simulink model "CSI_0313_4DC"  (R2018a)
settings: Solver=FixedStepDiscrete  StartTime=0.0  StopTime=Tstop  FixedStep=Tdelt  MaxStep=1e-4  RelTol=1e-3
values from neighbouring files (symbols this model uses):
  C = 12e-6    (= 1.2e-05)    [Inputparameter.m]
  Cdc = 4.76*10^-3    (= 0.00476)    [Inputparameter.m]
  Cemc = 1.5e-6    (= 1.5e-06)    [Inputparameter.m]
  fanalog = 7000    [Run.m]
  fKIUdc = 6    [Run.m]
  fKPUdc = 0.4    [Run.m]
  fTs = Update/18000    (= 0.000111111111111)    [Run.m]
  K120 = 0.0    (= 0)    [Run.m]
  K21 = 0.0    (= 0)    [Run.m]
  K5 = 0.0    (= 0)    [Run.m]
  K7 = 0.0    (= 0)    [Run.m]
  Kipll = 1.0    (= 1)    [Run.m]
  klmt = 0.3    [Run.m]
  Kpll = 20.0    (= 20)    [Run.m]
  Lgrid = 7.717e-4*10    (= 0.007717)    [Run.m]
  Lline = 60e-6    (= 6e-05)    [Inputparameter.m]
  Lpwm = 184.8e-6    (= 0.0001848)    [Inputparameter.m]
  mode = 1    [Run.m]
  Nsw = 18000/fbase    [Run.m]
  Qbpf = 1.0    (= 1)    [Run.m]
  Rc = 10e-3    (= 0.01)    [Inputparameter.m]
  Remc = 1e-3    (= 0.001)    [Inputparameter.m]
  Rgrid = 2*pi*fbase*Lgrid/XR    [Run.m]
  Rline = 4.95e-3    (= 0.00495)    [Inputparameter.m]
  Rpre = 2.2    [Inputparameter.m]
  Rpwm = 6.2e-3    (= 0.0062)    [Inputparameter.m]
  Tdelt = (fTs)/(200*Update)    (= 2.77777777778e-07)    [Run.m]
  Tdt = 1.27e-6    (= 1.27e-06)    [Run.m]
  tstart = 0.2    [Run.m]
  Tvstep = 1.5    [Run.m]
  Update = 2    [Run.m]
  Vbase = 400*sqrt(2/3)    [Inputparameter.m]
undefined symbols (not defined in the file or in its folder): sigbuilder_block
libraries: powerlib x412
(part 7 of 13)

== system CSI_0313_4DC/AIP9/Subsystem5/PLL ==
  Vabc : Inport
  ABC_To_RIZ : MATLAB Function  TreatAsAtomicUnit=on
  Constant : Constant  Value=2*pi*fFqBase  SampleTime=-1
  Constant1 : Constant  Value=2*pi
  Delay1 : Delay  DelayLength=1
  Delay2 : Delay  DelayLength=1
  Demux3 : Demux  Outputs=3
  Gain : Gain  Gain=1/(2*pi)
  Integral : MATLAB Function  TreatAsAtomicUnit=on  mask{fGain=1.0, fTs=fTs}
      mask prompts: fGain "Gain Value"; fTs "Sampling time [s]"
      mask help: Proportional Resonant Controller
  Math Function : Math  Operator=mod  SaturateOnIntegerOverflow=on
  PI Ctrl : MATLAB Function  TreatAsAtomicUnit=on  mask{fKP=fKPPLL, fKI=fKIPLL, fMinLmt=fDltMin, fMaxLmt=fDltMax, fTs=fTs}
      mask prompts: fKP "Proportional Gain"; fKI "Integral Coefficient"; fMinLmt "Minimum Limitation"; fMaxLmt "Maximum Limitation"; fTs "Sampling time [s]"
      mask help: Proportional Resonant Controller
  "Pos&Neg seq extract in subsystem " : Subsystem  mask{fQ=1.0, fTs=fTs}
      mask prompts: fQ "Quality Factor"; fTs "Sample Time"
  RIZ_To_DQ0 : MATLAB Function  TreatAsAtomicUnit=on  mask{iAxis=orient in A-axis}
      mask prompts: iAxis "Orient Axis Choice"
  Scope : Scope
  Sum : Sum  Inputs=++|
  Terminator : Terminator
  Terminator1 : Terminator
  f : Outport  VectorParamsAs1DForOutWhenUnconnected=on
  wt : Outport  Port=2  VectorParamsAs1DForOutWhenUnconnected=on
  VdPos : Outport  Port=3  VectorParamsAs1DForOutWhenUnconnected=on
  wires:
  [wt] -> wt/1
  ABC_To_RIZ/1(RIZ) -> [Vriz]
  [Vabc] -> ABC_To_RIZ/1(ABC)
  Delay2/1 -> RIZ_To_DQ0/2(wt)
  [wt] -> Delay2/1
  [f] -> f/1
  [VqPos] -> PI Ctrl/1(err)
  Math Function/1 -> [wt]
  Constant1/1 -> Math Function/2
  Integral/1(y) -> Math Function/1
  Vabc/1 -> [Vabc]
  Constant/1 -> Sum/1
  [VrizPos] -> RIZ_To_DQ0/1(RIZ)
  Sum/1 -> [w]
  PI Ctrl/1(y) -> Sum/2
  [Vdq0Pos] -> Demux3/1
  Demux3/1 -> [VdPos]
  Demux3/2 -> [VqPos]
  Gain/1 -> [f]
  [w] -> Integral/1(u)
  [w] -> Gain/1
  RIZ_To_DQ0/1(DQ0) -> [Vdq0Pos], Scope/1
  [Vriz] -> "Pos&Neg seq extract in subsystem "/1(RIZ)
  "Pos&Neg seq extract in subsystem "/1(RizPos) -> [VrizPos], VdPos/1
  "Pos&Neg seq extract in subsystem "/2(RizNeg) -> Terminator/1
  Demux3/3 -> Terminator1/1
  [f] -> Delay1/1
  "Pos&Neg seq extract in subsystem "/3(chk) -> [chk]
  Delay1/1 -> "Pos&Neg seq extract in subsystem "/2(ffc)

== system CSI_0313_4DC/AIP9/Subsystem7/BPF  ==
  Vriz : Inport
  Freq : Inport  Port=2
  Demux1 : Demux  Outputs=3
  IIR_BPF_Re1 : MATLAB Function  TreatAsAtomicUnit=on  mask{fQ=Qbpf, fTs=fTs, iMode=IIR2 used as BPF in SOGI}
      mask prompts: fQ "Quality factor"; fTs "Sample time [s]"; iMode "Modes of 2nd-order transfer function"
  IIR_BPF_Re2 : MATLAB Function  TreatAsAtomicUnit=on  mask{fQ=Qbpf, fTs=fTs, iMode=IIR2 used as BPF in SOGI}
      mask prompts: fQ "Quality factor"; fTs "Sample time [s]"; iMode "Modes of 2nd-order transfer function"
  IIR_BPF_Re3 : MATLAB Function  TreatAsAtomicUnit=on  mask{fQ=Qbpf, fTs=fTs, iMode=IIR2 used as BPF in SOGI}
      mask prompts: fQ "Quality factor"; fTs "Sample time [s]"; iMode "Modes of 2nd-order transfer function"
  Mux1 : Mux  Inputs=3
  VpccBPF : Outport  VectorParamsAs1DForOutWhenUnconnected=on
  wires:
  IIR_BPF_Re3/1(y) -> Mux1/3
  Demux1/3 -> IIR_BPF_Re3/1(u)
  IIR_BPF_Re1/1(y) -> Mux1/1
  Vriz/1 -> Demux1/1
  Demux1/2 -> IIR_BPF_Re2/1(u)
  IIR_BPF_Re2/1(y) -> Mux1/2
  Freq/1 -> IIR_BPF_Re1/2(fn), IIR_BPF_Re2/2(fn), IIR_BPF_Re3/2(fn)
  Mux1/1 -> VpccBPF/1
  Demux1/1 -> IIR_BPF_Re1/1(u)

== system CSI_0313_4DC/AIP9/Subsystem7/Pos Compensation1 ==
  Vdc : Inport
  wt : Inport  Port=2
  Constant3 : Constant  Value=0  SampleTime=-1
  DQ0_To_RIZ : MATLAB Function  TreatAsAtomicUnit=on  mask{iAxis=orient in A-axis}
      mask prompts: iAxis "Orient Axis Choice"
  Gain2 : Gain  Gain=1/Vbase
  Gain3 : Gain  Gain=1/Vbase
  Gain4 : Gain  Gain=-1
  Ground : Ground
  Mux : Mux  Inputs=3
  PI Ctrl2 : MATLAB Function  TreatAsAtomicUnit=on  mask{fKP=fKPUdc, fKI=fKIUdc, fMinLmt=-klmt*Vbase, fMaxLmt=klmt*Vbase, fTs=fTs}
      mask prompts: fKP "Proportional Gain"; fKI "Integral Coefficient"; fMinLmt "Minimum Limitation"; fMaxLmt "Maximum Limitation"; fTs "Sampling time [s]"
      mask help: Proportional Resonant Controller
  RIZ_To_ABC : MATLAB Function  TreatAsAtomicUnit=on
  RIZ_To_DQ0 : MATLAB Function  TreatAsAtomicUnit=on  mask{iAxis=orient in A-axis}
      mask prompts: iAxis "Orient Axis Choice"
  Scope : Scope
  Scope1 : Scope
  Scope2 : Scope
  Scope6 : Scope  NumInputPorts=2
  Step : Step  Time=Tvstep  Before=650  After=700
  Sum1 : Sum  Inputs=|-+
  VabcFBPU : Outport
  wires:
  Constant3/1 -> Mux/1
  [VdRef] -> Gain4/1, Mux/2
  Gain3/1 -> Scope2/1
  RIZ_To_DQ0/1(DQ0) -> Gain3/1
  Step/1 -> Sum1/1, Scope6/1
  Gain2/1 -> VabcFBPU/1
  DQ0_To_RIZ/1(RIZ) -> RIZ_To_ABC/1(RIZ), RIZ_To_DQ0/1(RIZ)
  RIZ_To_ABC/1(ABC) -> [VabcFB]
  wt/1 -> DQ0_To_RIZ/2(wt), RIZ_To_DQ0/2(wt)
  Mux/1 -> DQ0_To_RIZ/1(DQ0)
  Ground/1 -> Mux/3
  [VdRef] -> Scope/1
  [VabcFB] -> Gain2/1, Scope1/1
  Vdc/1 -> [Vdc]
  Sum1/1 -> PI Ctrl2/1(err)
  PI Ctrl2/1(y) -> [VdRef]
  [Vdc] -> Scope6/2, Sum1/2

== system CSI_0313_4DC/AIP9/Subsystem7/Subsystem5 ==
  Vabc : Inport
  Vdc : Inport  Port=2
  3rd Injection1 : MATLAB Function  TreatAsAtomicUnit=on  mask{mode=mode}
      mask prompts: mode "Three wire/four wire"
  Vmod : Outport  VectorParamsAs1DForOutWhenUnconnected=on
  wires:
  Vdc/1 -> 3rd Injection1/2(Vdc)
  3rd Injection1/1(Mod) -> Vmod/1
  Vabc/1 -> 3rd Injection1/1(Vabc)

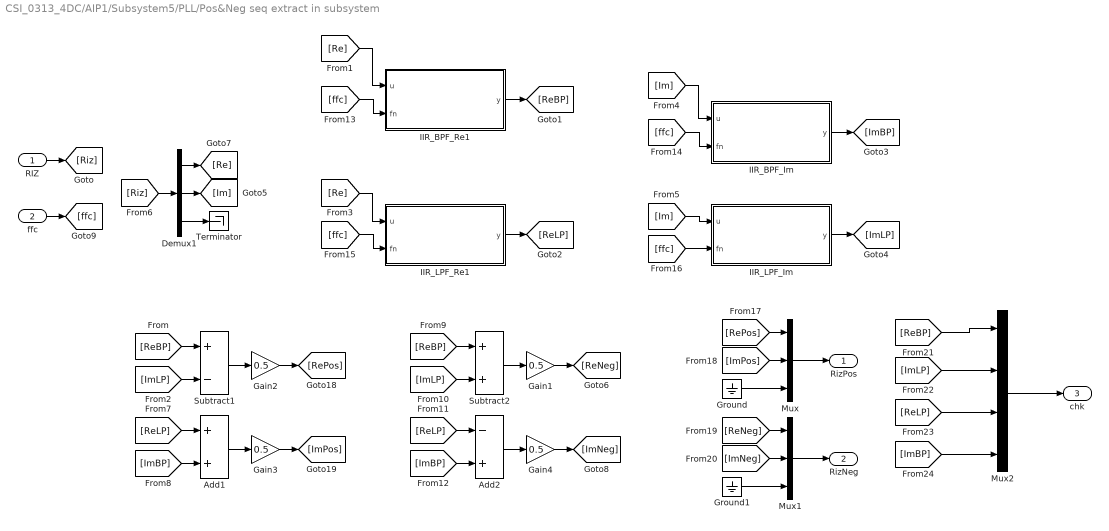
== system CSI_0313_4DC/AIP1/Subsystem5/PLL/Pos&Neg seq extract in subsystem  ==
  RIZ : Inport
  ffc : Inport  Port=2
  Add1 : Sum
  Add2 : Sum  Inputs=-+
  Demux1 : Demux  Outputs=3
  Gain{1..4} (4 alike) : Gain  Gain=0.5
  Ground : Ground
  Ground1 : Ground
  IIR_BPF_Im : MATLAB Function  TreatAsAtomicUnit=on  mask{fQ=fQ, fTs=fTs, iMode=IIR2 used as BPF in SOGI}
      mask prompts: fQ "Quality factor"; fTs "Sample time [s]"; iMode "Modes of 2nd-order transfer function"
  IIR_BPF_Re1 : MATLAB Function  TreatAsAtomicUnit=on  mask{fQ=fQ, fTs=fTs, iMode=IIR2 used as BPF in SOGI}
      mask prompts: fQ "Quality factor"; fTs "Sample time [s]"; iMode "Modes of 2nd-order transfer function"
  IIR_LPF_Im : MATLAB Function  TreatAsAtomicUnit=on  mask{fQ=fQ, fTs=fTs, iMode=IIR2 used as LPF in SOGI}
      mask prompts: fQ "Quality factor"; fTs "Sample time [s]"; iMode "Modes of 2nd-order transfer function"
  IIR_LPF_Re1 : MATLAB Function  TreatAsAtomicUnit=on  mask{fQ=fQ, fTs=fTs, iMode=IIR2 used as LPF in SOGI}
      mask prompts: fQ "Quality factor"; fTs "Sample time [s]"; iMode "Modes of 2nd-order transfer function"
  Mux : Mux  Inputs=3
  Mux1 : Mux  Inputs=3
  Mux2 : Mux
  Subtract1 : Sum  Inputs=+-
  Subtract2 : Sum
  Terminator : Terminator
  RizPos : Outport  VectorParamsAs1DForOutWhenUnconnected=on
  RizNeg : Outport  Port=2  VectorParamsAs1DForOutWhenUnconnected=on
  chk : Outport  Port=3  VectorParamsAs1DForOutWhenUnconnected=on
  wires:
  [ImBP] -> Add2/2
  [ffc] -> IIR_BPF_Im/2(fn)
  Add1/1 -> Gain3/1
  [ReLP] -> Mux2/3
  [ImBP] -> Mux2/4
  Demux1/1 -> [Re]
  RIZ/1 -> [Riz]
  Ground1/1 -> Mux1/3
  [ImLP] -> Mux2/2
  Add2/1 -> Gain4/1
  [ImLP] -> Subtract1/2
  [ReLP] -> Add1/1
  [ReBP] -> Subtract2/1
  [ImBP] -> Add1/2
  Gain1/1 -> [ReNeg]
  IIR_LPF_Re1/1(y) -> [ReLP]
  [Re] -> IIR_BPF_Re1/1(u)
  [RePos] -> Mux/1
  [ReBP] -> Subtract1/1
  Mux/1 -> RizPos/1
  [ffc] -> IIR_BPF_Re1/2(fn)
  Mux1/1 -> RizNeg/1
  IIR_BPF_Im/1(y) -> [ImBP]
  [Im] -> IIR_BPF_Im/1(u)
  Demux1/3 -> Terminator/1
  IIR_BPF_Re1/1(y) -> [ReBP]
  Gain3/1 -> [ImPos]
  IIR_LPF_Im/1(y) -> [ImLP]
  [ImNeg] -> Mux1/2
  [Im] -> IIR_LPF_Im/1(u)
  [ffc] -> IIR_LPF_Im/2(fn)
  [ImLP] -> Subtract2/2
  Demux1/2 -> [Im]
  Subtract1/1 -> Gain2/1
  [Re] -> IIR_LPF_Re1/1(u)
  [ffc] -> IIR_LPF_Re1/2(fn)
  [ReBP] -> Mux2/1
  [Riz] -> Demux1/1
  Ground/1 -> Mux/3
  [ReNeg] -> Mux1/1
  Mux2/1 -> chk/1
  Gain4/1 -> [ImNeg]
  Subtract2/1 -> Gain1/1
  Gain2/1 -> [RePos]
  [ReLP] -> Add2/1
  ffc/1 -> [ffc]
  [ImPos] -> Mux/2

== system CSI_0313_4DC/AIP10/Subsystem5/PLL/Pos&Neg seq extract in subsystem  ==
  RIZ : Inport
  ffc : Inport  Port=2
  Add1 : Sum
  Add2 : Sum  Inputs=-+
  Demux1 : Demux  Outputs=3
  Gain{1..4} (4 alike) : Gain  Gain=0.5
  Ground : Ground
  Ground1 : Ground
  IIR_BPF_Im : MATLAB Function  TreatAsAtomicUnit=on  mask{fQ=fQ, fTs=fTs, iMode=IIR2 used as BPF in SOGI}
      mask prompts: fQ "Quality factor"; fTs "Sample time [s]"; iMode "Modes of 2nd-order transfer function"
  IIR_BPF_Re1 : MATLAB Function  TreatAsAtomicUnit=on  mask{fQ=fQ, fTs=fTs, iMode=IIR2 used as BPF in SOGI}
      mask prompts: fQ "Quality factor"; fTs "Sample time [s]"; iMode "Modes of 2nd-order transfer function"
  IIR_LPF_Im : MATLAB Function  TreatAsAtomicUnit=on  mask{fQ=fQ, fTs=fTs, iMode=IIR2 used as LPF in SOGI}
      mask prompts: fQ "Quality factor"; fTs "Sample time [s]"; iMode "Modes of 2nd-order transfer function"
  IIR_LPF_Re1 : MATLAB Function  TreatAsAtomicUnit=on  mask{fQ=fQ, fTs=fTs, iMode=IIR2 used as LPF in SOGI}
      mask prompts: fQ "Quality factor"; fTs "Sample time [s]"; iMode "Modes of 2nd-order transfer function"
  Mux : Mux  Inputs=3
  Mux1 : Mux  Inputs=3
  Mux2 : Mux
  Subtract1 : Sum  Inputs=+-
  Subtract2 : Sum
  Terminator : Terminator
  RizPos : Outport  VectorParamsAs1DForOutWhenUnconnected=on
  RizNeg : Outport  Port=2  VectorParamsAs1DForOutWhenUnconnected=on
  chk : Outport  Port=3  VectorParamsAs1DForOutWhenUnconnected=on
  wires:
  [ImBP] -> Add2/2
  [ffc] -> IIR_BPF_Im/2(fn)
  Add1/1 -> Gain3/1
  [ReLP] -> Mux2/3
  [ImBP] -> Mux2/4
  Demux1/1 -> [Re]
  RIZ/1 -> [Riz]
  Ground1/1 -> Mux1/3
  [ImLP] -> Mux2/2
  Add2/1 -> Gain4/1
  [ImLP] -> Subtract1/2
  [ReLP] -> Add1/1
  [ReBP] -> Subtract2/1
  [ImBP] -> Add1/2
  Gain1/1 -> [ReNeg]
  IIR_LPF_Re1/1(y) -> [ReLP]
  [Re] -> IIR_BPF_Re1/1(u)
  [RePos] -> Mux/1
  [ReBP] -> Subtract1/1
  Mux/1 -> RizPos/1
  [ffc] -> IIR_BPF_Re1/2(fn)
  Mux1/1 -> RizNeg/1
  IIR_BPF_Im/1(y) -> [ImBP]
  [Im] -> IIR_BPF_Im/1(u)
  Demux1/3 -> Terminator/1
  IIR_BPF_Re1/1(y) -> [ReBP]
  Gain3/1 -> [ImPos]
  IIR_LPF_Im/1(y) -> [ImLP]
  [ImNeg] -> Mux1/2
  [Im] -> IIR_LPF_Im/1(u)
  [ffc] -> IIR_LPF_Im/2(fn)
  [ImLP] -> Subtract2/2
  Demux1/2 -> [Im]
  Subtract1/1 -> Gain2/1
  [Re] -> IIR_LPF_Re1/1(u)
  [ffc] -> IIR_LPF_Re1/2(fn)
  [ReBP] -> Mux2/1
  [Riz] -> Demux1/1
  Ground/1 -> Mux/3
  [ReNeg] -> Mux1/1
  Mux2/1 -> chk/1
  Gain4/1 -> [ImNeg]
  Subtract2/1 -> Gain1/1
  Gain2/1 -> [RePos]
  [ReLP] -> Add2/1
  ffc/1 -> [ffc]
  [ImPos] -> Mux/2

== system CSI_0313_4DC/AIP2/Subsystem5/PLL/Pos&Neg seq extract in subsystem  ==
  RIZ : Inport
  ffc : Inport  Port=2
  Add1 : Sum
  Add2 : Sum  Inputs=-+
  Demux1 : Demux  Outputs=3
  Gain{1..4} (4 alike) : Gain  Gain=0.5
  Ground : Ground
  Ground1 : Ground
  IIR_BPF_Im : MATLAB Function  TreatAsAtomicUnit=on  mask{fQ=fQ, fTs=fTs, iMode=IIR2 used as BPF in SOGI}
      mask prompts: fQ "Quality factor"; fTs "Sample time [s]"; iMode "Modes of 2nd-order transfer function"
  IIR_BPF_Re1 : MATLAB Function  TreatAsAtomicUnit=on  mask{fQ=fQ, fTs=fTs, iMode=IIR2 used as BPF in SOGI}
      mask prompts: fQ "Quality factor"; fTs "Sample time [s]"; iMode "Modes of 2nd-order transfer function"
  IIR_LPF_Im : MATLAB Function  TreatAsAtomicUnit=on  mask{fQ=fQ, fTs=fTs, iMode=IIR2 used as LPF in SOGI}
      mask prompts: fQ "Quality factor"; fTs "Sample time [s]"; iMode "Modes of 2nd-order transfer function"
  IIR_LPF_Re1 : MATLAB Function  TreatAsAtomicUnit=on  mask{fQ=fQ, fTs=fTs, iMode=IIR2 used as LPF in SOGI}
      mask prompts: fQ "Quality factor"; fTs "Sample time [s]"; iMode "Modes of 2nd-order transfer function"
  Mux : Mux  Inputs=3
  Mux1 : Mux  Inputs=3
  Mux2 : Mux
  Subtract1 : Sum  Inputs=+-
  Subtract2 : Sum
  Terminator : Terminator
  RizPos : Outport  VectorParamsAs1DForOutWhenUnconnected=on
  RizNeg : Outport  Port=2  VectorParamsAs1DForOutWhenUnconnected=on
  chk : Outport  Port=3  VectorParamsAs1DForOutWhenUnconnected=on
  wires:
  [ImPos] -> Mux/2
  ffc/1 -> [ffc]
  [ReLP] -> Add2/1
  Gain2/1 -> [RePos]
  Subtract2/1 -> Gain1/1
  Gain4/1 -> [ImNeg]
  Mux2/1 -> chk/1
  [ReNeg] -> Mux1/1
  Ground/1 -> Mux/3
  [Riz] -> Demux1/1
  [ReBP] -> Mux2/1
  [ffc] -> IIR_LPF_Re1/2(fn)
  [Re] -> IIR_LPF_Re1/1(u)
  Subtract1/1 -> Gain2/1
  Demux1/2 -> [Im]
  [ImLP] -> Subtract2/2
  [ffc] -> IIR_LPF_Im/2(fn)
  [Im] -> IIR_LPF_Im/1(u)
  [ImNeg] -> Mux1/2
  IIR_LPF_Im/1(y) -> [ImLP]
  Gain3/1 -> [ImPos]
  IIR_BPF_Re1/1(y) -> [ReBP]
  Demux1/3 -> Terminator/1
  [Im] -> IIR_BPF_Im/1(u)
  IIR_BPF_Im/1(y) -> [ImBP]
  Mux1/1 -> RizNeg/1
  [ffc] -> IIR_BPF_Re1/2(fn)
  Mux/1 -> RizPos/1
  [ReBP] -> Subtract1/1
  [RePos] -> Mux/1
  [Re] -> IIR_BPF_Re1/1(u)
  IIR_LPF_Re1/1(y) -> [ReLP]
  Gain1/1 -> [ReNeg]
  [ImBP] -> Add1/2
  [ReBP] -> Subtract2/1
  [ReLP] -> Add1/1
  [ImLP] -> Subtract1/2
  Add2/1 -> Gain4/1
  [ImLP] -> Mux2/2
  Ground1/1 -> Mux1/3
  RIZ/1 -> [Riz]
  Demux1/1 -> [Re]
  [ImBP] -> Mux2/4
  [ReLP] -> Mux2/3
  Add1/1 -> Gain3/1
  [ffc] -> IIR_BPF_Im/2(fn)
  [ImBP] -> Add2/2

== system CSI_0313_4DC/AIP3/Subsystem5/PLL/Pos&Neg seq extract in subsystem  ==
  RIZ : Inport
  ffc : Inport  Port=2
  Add1 : Sum
  Add2 : Sum  Inputs=-+
  Demux1 : Demux  Outputs=3
  Gain{1..4} (4 alike) : Gain  Gain=0.5
  Ground : Ground
  Ground1 : Ground
  IIR_BPF_Im : MATLAB Function  TreatAsAtomicUnit=on  mask{fQ=fQ, fTs=fTs, iMode=IIR2 used as BPF in SOGI}
      mask prompts: fQ "Quality factor"; fTs "Sample time [s]"; iMode "Modes of 2nd-order transfer function"
  IIR_BPF_Re1 : MATLAB Function  TreatAsAtomicUnit=on  mask{fQ=fQ, fTs=fTs, iMode=IIR2 used as BPF in SOGI}
      mask prompts: fQ "Quality factor"; fTs "Sample time [s]"; iMode "Modes of 2nd-order transfer function"
  IIR_LPF_Im : MATLAB Function  TreatAsAtomicUnit=on  mask{fQ=fQ, fTs=fTs, iMode=IIR2 used as LPF in SOGI}
      mask prompts: fQ "Quality factor"; fTs "Sample time [s]"; iMode "Modes of 2nd-order transfer function"
  IIR_LPF_Re1 : MATLAB Function  TreatAsAtomicUnit=on  mask{fQ=fQ, fTs=fTs, iMode=IIR2 used as LPF in SOGI}
      mask prompts: fQ "Quality factor"; fTs "Sample time [s]"; iMode "Modes of 2nd-order transfer function"
  Mux : Mux  Inputs=3
  Mux1 : Mux  Inputs=3
  Mux2 : Mux
  Subtract1 : Sum  Inputs=+-
  Subtract2 : Sum
  Terminator : Terminator
  RizPos : Outport  VectorParamsAs1DForOutWhenUnconnected=on
  RizNeg : Outport  Port=2  VectorParamsAs1DForOutWhenUnconnected=on
  chk : Outport  Port=3  VectorParamsAs1DForOutWhenUnconnected=on
  wires:
  [ImBP] -> Add2/2
  [ffc] -> IIR_BPF_Im/2(fn)
  Add1/1 -> Gain3/1
  [ReLP] -> Mux2/3
  [ImBP] -> Mux2/4
  Demux1/1 -> [Re]
  RIZ/1 -> [Riz]
  Ground1/1 -> Mux1/3
  [ImLP] -> Mux2/2
  Add2/1 -> Gain4/1
  [ImLP] -> Subtract1/2
  [ReLP] -> Add1/1
  [ReBP] -> Subtract2/1
  [ImBP] -> Add1/2
  Gain1/1 -> [ReNeg]
  IIR_LPF_Re1/1(y) -> [ReLP]
  [Re] -> IIR_BPF_Re1/1(u)
  [RePos] -> Mux/1
  [ReBP] -> Subtract1/1
  Mux/1 -> RizPos/1
  [ffc] -> IIR_BPF_Re1/2(fn)
  Mux1/1 -> RizNeg/1
  IIR_BPF_Im/1(y) -> [ImBP]
  [Im] -> IIR_BPF_Im/1(u)
  Demux1/3 -> Terminator/1
  IIR_BPF_Re1/1(y) -> [ReBP]
  Gain3/1 -> [ImPos]
  IIR_LPF_Im/1(y) -> [ImLP]
  [ImNeg] -> Mux1/2
  [Im] -> IIR_LPF_Im/1(u)
  [ffc] -> IIR_LPF_Im/2(fn)
  [ImLP] -> Subtract2/2
  Demux1/2 -> [Im]
  Subtract1/1 -> Gain2/1
  [Re] -> IIR_LPF_Re1/1(u)
  [ffc] -> IIR_LPF_Re1/2(fn)
  [ReBP] -> Mux2/1
  [Riz] -> Demux1/1
  Ground/1 -> Mux/3
  [ReNeg] -> Mux1/1
  Mux2/1 -> chk/1
  Gain4/1 -> [ImNeg]
  Subtract2/1 -> Gain1/1
  Gain2/1 -> [RePos]
  [ReLP] -> Add2/1
  ffc/1 -> [ffc]
  [ImPos] -> Mux/2

== system CSI_0313_4DC/AIP4/Subsystem5/PLL/Pos&Neg seq extract in subsystem  ==
  RIZ : Inport
  ffc : Inport  Port=2
  Add1 : Sum
  Add2 : Sum  Inputs=-+
  Demux1 : Demux  Outputs=3
  Gain{1..4} (4 alike) : Gain  Gain=0.5
  Ground : Ground
  Ground1 : Ground
  IIR_BPF_Im : MATLAB Function  TreatAsAtomicUnit=on  mask{fQ=fQ, fTs=fTs, iMode=IIR2 used as BPF in SOGI}
      mask prompts: fQ "Quality factor"; fTs "Sample time [s]"; iMode "Modes of 2nd-order transfer function"
  IIR_BPF_Re1 : MATLAB Function  TreatAsAtomicUnit=on  mask{fQ=fQ, fTs=fTs, iMode=IIR2 used as BPF in SOGI}
      mask prompts: fQ "Quality factor"; fTs "Sample time [s]"; iMode "Modes of 2nd-order transfer function"
  IIR_LPF_Im : MATLAB Function  TreatAsAtomicUnit=on  mask{fQ=fQ, fTs=fTs, iMode=IIR2 used as LPF in SOGI}
      mask prompts: fQ "Quality factor"; fTs "Sample time [s]"; iMode "Modes of 2nd-order transfer function"
  IIR_LPF_Re1 : MATLAB Function  TreatAsAtomicUnit=on  mask{fQ=fQ, fTs=fTs, iMode=IIR2 used as LPF in SOGI}
      mask prompts: fQ "Quality factor"; fTs "Sample time [s]"; iMode "Modes of 2nd-order transfer function"
  Mux : Mux  Inputs=3
  Mux1 : Mux  Inputs=3
  Mux2 : Mux
  Subtract1 : Sum  Inputs=+-
  Subtract2 : Sum
  Terminator : Terminator
  RizPos : Outport  VectorParamsAs1DForOutWhenUnconnected=on
  RizNeg : Outport  Port=2  VectorParamsAs1DForOutWhenUnconnected=on
  chk : Outport  Port=3  VectorParamsAs1DForOutWhenUnconnected=on
  wires:
  [ImPos] -> Mux/2
  ffc/1 -> [ffc]
  [ReLP] -> Add2/1
  Gain2/1 -> [RePos]
  Subtract2/1 -> Gain1/1
  Gain4/1 -> [ImNeg]
  Mux2/1 -> chk/1
  [ReNeg] -> Mux1/1
  Ground/1 -> Mux/3
  [Riz] -> Demux1/1
  [ReBP] -> Mux2/1
  [ffc] -> IIR_LPF_Re1/2(fn)
  [Re] -> IIR_LPF_Re1/1(u)
  Subtract1/1 -> Gain2/1
  Demux1/2 -> [Im]
  [ImLP] -> Subtract2/2
  [ffc] -> IIR_LPF_Im/2(fn)
  [Im] -> IIR_LPF_Im/1(u)
  [ImNeg] -> Mux1/2
  IIR_LPF_Im/1(y) -> [ImLP]
  Gain3/1 -> [ImPos]
  IIR_BPF_Re1/1(y) -> [ReBP]
  Demux1/3 -> Terminator/1
  [Im] -> IIR_BPF_Im/1(u)
  IIR_BPF_Im/1(y) -> [ImBP]
  Mux1/1 -> RizNeg/1
  [ffc] -> IIR_BPF_Re1/2(fn)
  Mux/1 -> RizPos/1
  [ReBP] -> Subtract1/1
  [RePos] -> Mux/1
  [Re] -> IIR_BPF_Re1/1(u)
  IIR_LPF_Re1/1(y) -> [ReLP]
  Gain1/1 -> [ReNeg]
  [ImBP] -> Add1/2
  [ReBP] -> Subtract2/1
  [ReLP] -> Add1/1
  [ImLP] -> Subtract1/2
  Add2/1 -> Gain4/1
  [ImLP] -> Mux2/2
  Ground1/1 -> Mux1/3
  RIZ/1 -> [Riz]
  Demux1/1 -> [Re]
  [ImBP] -> Mux2/4
  [ReLP] -> Mux2/3
  Add1/1 -> Gain3/1
  [ffc] -> IIR_BPF_Im/2(fn)
  [ImBP] -> Add2/2

== system CSI_0313_4DC/AIP5/Subsystem5/PLL/Pos&Neg seq extract in subsystem  ==
  RIZ : Inport
  ffc : Inport  Port=2
  Add1 : Sum
  Add2 : Sum  Inputs=-+
  Demux1 : Demux  Outputs=3
  Gain{1..4} (4 alike) : Gain  Gain=0.5
  Ground : Ground
  Ground1 : Ground
  IIR_BPF_Im : MATLAB Function  TreatAsAtomicUnit=on  mask{fQ=fQ, fTs=fTs, iMode=IIR2 used as BPF in SOGI}
      mask prompts: fQ "Quality factor"; fTs "Sample time [s]"; iMode "Modes of 2nd-order transfer function"
  IIR_BPF_Re1 : MATLAB Function  TreatAsAtomicUnit=on  mask{fQ=fQ, fTs=fTs, iMode=IIR2 used as BPF in SOGI}
      mask prompts: fQ "Quality factor"; fTs "Sample time [s]"; iMode "Modes of 2nd-order transfer function"
  IIR_LPF_Im : MATLAB Function  TreatAsAtomicUnit=on  mask{fQ=fQ, fTs=fTs, iMode=IIR2 used as LPF in SOGI}
      mask prompts: fQ "Quality factor"; fTs "Sample time [s]"; iMode "Modes of 2nd-order transfer function"
  IIR_LPF_Re1 : MATLAB Function  TreatAsAtomicUnit=on  mask{fQ=fQ, fTs=fTs, iMode=IIR2 used as LPF in SOGI}
      mask prompts: fQ "Quality factor"; fTs "Sample time [s]"; iMode "Modes of 2nd-order transfer function"
  Mux : Mux  Inputs=3
  Mux1 : Mux  Inputs=3
  Mux2 : Mux
  Subtract1 : Sum  Inputs=+-
  Subtract2 : Sum
  Terminator : Terminator
  RizPos : Outport  VectorParamsAs1DForOutWhenUnconnected=on
  RizNeg : Outport  Port=2  VectorParamsAs1DForOutWhenUnconnected=on
  chk : Outport  Port=3  VectorParamsAs1DForOutWhenUnconnected=on
  wires:
  [ImBP] -> Add2/2
  [ffc] -> IIR_BPF_Im/2(fn)
  Add1/1 -> Gain3/1
  [ReLP] -> Mux2/3
  [ImBP] -> Mux2/4
  Demux1/1 -> [Re]
  RIZ/1 -> [Riz]
  Ground1/1 -> Mux1/3
  [ImLP] -> Mux2/2
  Add2/1 -> Gain4/1
  [ImLP] -> Subtract1/2
  [ReLP] -> Add1/1
  [ReBP] -> Subtract2/1
  [ImBP] -> Add1/2
  Gain1/1 -> [ReNeg]
  IIR_LPF_Re1/1(y) -> [ReLP]
  [Re] -> IIR_BPF_Re1/1(u)
  [RePos] -> Mux/1
  [ReBP] -> Subtract1/1
  Mux/1 -> RizPos/1
  [ffc] -> IIR_BPF_Re1/2(fn)
  Mux1/1 -> RizNeg/1
  IIR_BPF_Im/1(y) -> [ImBP]
  [Im] -> IIR_BPF_Im/1(u)
  Demux1/3 -> Terminator/1
  IIR_BPF_Re1/1(y) -> [ReBP]
  Gain3/1 -> [ImPos]
  IIR_LPF_Im/1(y) -> [ImLP]
  [ImNeg] -> Mux1/2
  [Im] -> IIR_LPF_Im/1(u)
  [ffc] -> IIR_LPF_Im/2(fn)
  [ImLP] -> Subtract2/2
  Demux1/2 -> [Im]
  Subtract1/1 -> Gain2/1
  [Re] -> IIR_LPF_Re1/1(u)
  [ffc] -> IIR_LPF_Re1/2(fn)
  [ReBP] -> Mux2/1
  [Riz] -> Demux1/1
  Ground/1 -> Mux/3
  [ReNeg] -> Mux1/1
  Mux2/1 -> chk/1
  Gain4/1 -> [ImNeg]
  Subtract2/1 -> Gain1/1
  Gain2/1 -> [RePos]
  [ReLP] -> Add2/1
  ffc/1 -> [ffc]
  [ImPos] -> Mux/2

== system CSI_0313_4DC/AIP6/Subsystem5/PLL/Pos&Neg seq extract in subsystem  ==
  RIZ : Inport
  ffc : Inport  Port=2
  Add1 : Sum
  Add2 : Sum  Inputs=-+
  Demux1 : Demux  Outputs=3
  Gain{1..4} (4 alike) : Gain  Gain=0.5
  Ground : Ground
  Ground1 : Ground
  IIR_BPF_Im : MATLAB Function  TreatAsAtomicUnit=on  mask{fQ=fQ, fTs=fTs, iMode=IIR2 used as BPF in SOGI}
      mask prompts: fQ "Quality factor"; fTs "Sample time [s]"; iMode "Modes of 2nd-order transfer function"
  IIR_BPF_Re1 : MATLAB Function  TreatAsAtomicUnit=on  mask{fQ=fQ, fTs=fTs, iMode=IIR2 used as BPF in SOGI}
      mask prompts: fQ "Quality factor"; fTs "Sample time [s]"; iMode "Modes of 2nd-order transfer function"
  IIR_LPF_Im : MATLAB Function  TreatAsAtomicUnit=on  mask{fQ=fQ, fTs=fTs, iMode=IIR2 used as LPF in SOGI}
      mask prompts: fQ "Quality factor"; fTs "Sample time [s]"; iMode "Modes of 2nd-order transfer function"
  IIR_LPF_Re1 : MATLAB Function  TreatAsAtomicUnit=on  mask{fQ=fQ, fTs=fTs, iMode=IIR2 used as LPF in SOGI}
      mask prompts: fQ "Quality factor"; fTs "Sample time [s]"; iMode "Modes of 2nd-order transfer function"
  Mux : Mux  Inputs=3
  Mux1 : Mux  Inputs=3
  Mux2 : Mux
  Subtract1 : Sum  Inputs=+-
  Subtract2 : Sum
  Terminator : Terminator
  RizPos : Outport  VectorParamsAs1DForOutWhenUnconnected=on
  RizNeg : Outport  Port=2  VectorParamsAs1DForOutWhenUnconnected=on
  chk : Outport  Port=3  VectorParamsAs1DForOutWhenUnconnected=on
  wires:
  [ImBP] -> Add2/2
  [ffc] -> IIR_BPF_Im/2(fn)
  Add1/1 -> Gain3/1
  [ReLP] -> Mux2/3
  [ImBP] -> Mux2/4
  Demux1/1 -> [Re]
  RIZ/1 -> [Riz]
  Ground1/1 -> Mux1/3
  [ImLP] -> Mux2/2
  Add2/1 -> Gain4/1
  [ImLP] -> Subtract1/2
  [ReLP] -> Add1/1
  [ReBP] -> Subtract2/1
  [ImBP] -> Add1/2
  Gain1/1 -> [ReNeg]
  IIR_LPF_Re1/1(y) -> [ReLP]
  [Re] -> IIR_BPF_Re1/1(u)
  [RePos] -> Mux/1
  [ReBP] -> Subtract1/1
  Mux/1 -> RizPos/1
  [ffc] -> IIR_BPF_Re1/2(fn)
  Mux1/1 -> RizNeg/1
  IIR_BPF_Im/1(y) -> [ImBP]
  [Im] -> IIR_BPF_Im/1(u)
  Demux1/3 -> Terminator/1
  IIR_BPF_Re1/1(y) -> [ReBP]
  Gain3/1 -> [ImPos]
  IIR_LPF_Im/1(y) -> [ImLP]
  [ImNeg] -> Mux1/2
  [Im] -> IIR_LPF_Im/1(u)
  [ffc] -> IIR_LPF_Im/2(fn)
  [ImLP] -> Subtract2/2
  Demux1/2 -> [Im]
  Subtract1/1 -> Gain2/1
  [Re] -> IIR_LPF_Re1/1(u)
  [ffc] -> IIR_LPF_Re1/2(fn)
  [ReBP] -> Mux2/1
  [Riz] -> Demux1/1
  Ground/1 -> Mux/3
  [ReNeg] -> Mux1/1
  Mux2/1 -> chk/1
  Gain4/1 -> [ImNeg]
  Subtract2/1 -> Gain1/1
  Gain2/1 -> [RePos]
  [ReLP] -> Add2/1
  ffc/1 -> [ffc]
  [ImPos] -> Mux/2

== system CSI_0313_4DC/AIP7/Subsystem5/PLL/Pos&Neg seq extract in subsystem  ==
  RIZ : Inport
  ffc : Inport  Port=2
  Add1 : Sum
  Add2 : Sum  Inputs=-+
  Demux1 : Demux  Outputs=3
  Gain{1..4} (4 alike) : Gain  Gain=0.5
  Ground : Ground
  Ground1 : Ground
  IIR_BPF_Im : MATLAB Function  TreatAsAtomicUnit=on  mask{fQ=fQ, fTs=fTs, iMode=IIR2 used as BPF in SOGI}
      mask prompts: fQ "Quality factor"; fTs "Sample time [s]"; iMode "Modes of 2nd-order transfer function"
  IIR_BPF_Re1 : MATLAB Function  TreatAsAtomicUnit=on  mask{fQ=fQ, fTs=fTs, iMode=IIR2 used as BPF in SOGI}
      mask prompts: fQ "Quality factor"; fTs "Sample time [s]"; iMode "Modes of 2nd-order transfer function"
  IIR_LPF_Im : MATLAB Function  TreatAsAtomicUnit=on  mask{fQ=fQ, fTs=fTs, iMode=IIR2 used as LPF in SOGI}
      mask prompts: fQ "Quality factor"; fTs "Sample time [s]"; iMode "Modes of 2nd-order transfer function"
  IIR_LPF_Re1 : MATLAB Function  TreatAsAtomicUnit=on  mask{fQ=fQ, fTs=fTs, iMode=IIR2 used as LPF in SOGI}
      mask prompts: fQ "Quality factor"; fTs "Sample time [s]"; iMode "Modes of 2nd-order transfer function"
  Mux : Mux  Inputs=3
  Mux1 : Mux  Inputs=3
  Mux2 : Mux
  Subtract1 : Sum  Inputs=+-
  Subtract2 : Sum
  Terminator : Terminator
  RizPos : Outport  VectorParamsAs1DForOutWhenUnconnected=on
  RizNeg : Outport  Port=2  VectorParamsAs1DForOutWhenUnconnected=on
  chk : Outport  Port=3  VectorParamsAs1DForOutWhenUnconnected=on
  wires:
  [ImPos] -> Mux/2
  ffc/1 -> [ffc]
  [ReLP] -> Add2/1
  Gain2/1 -> [RePos]
  Subtract2/1 -> Gain1/1
  Gain4/1 -> [ImNeg]
  Mux2/1 -> chk/1
  [ReNeg] -> Mux1/1
  Ground/1 -> Mux/3
  [Riz] -> Demux1/1
  [ReBP] -> Mux2/1
  [ffc] -> IIR_LPF_Re1/2(fn)
  [Re] -> IIR_LPF_Re1/1(u)
  Subtract1/1 -> Gain2/1
  Demux1/2 -> [Im]
  [ImLP] -> Subtract2/2
  [ffc] -> IIR_LPF_Im/2(fn)
  [Im] -> IIR_LPF_Im/1(u)
  [ImNeg] -> Mux1/2
  IIR_LPF_Im/1(y) -> [ImLP]
  Gain3/1 -> [ImPos]
  IIR_BPF_Re1/1(y) -> [ReBP]
  Demux1/3 -> Terminator/1
  [Im] -> IIR_BPF_Im/1(u)
  IIR_BPF_Im/1(y) -> [ImBP]
  Mux1/1 -> RizNeg/1
  [ffc] -> IIR_BPF_Re1/2(fn)
  Mux/1 -> RizPos/1
  [ReBP] -> Subtract1/1
  [RePos] -> Mux/1
  [Re] -> IIR_BPF_Re1/1(u)
  IIR_LPF_Re1/1(y) -> [ReLP]
  Gain1/1 -> [ReNeg]
  [ImBP] -> Add1/2
  [ReBP] -> Subtract2/1
  [ReLP] -> Add1/1
  [ImLP] -> Subtract1/2
  Add2/1 -> Gain4/1
  [ImLP] -> Mux2/2
  Ground1/1 -> Mux1/3
  RIZ/1 -> [Riz]
  Demux1/1 -> [Re]
  [ImBP] -> Mux2/4
  [ReLP] -> Mux2/3
  Add1/1 -> Gain3/1
  [ffc] -> IIR_BPF_Im/2(fn)
  [ImBP] -> Add2/2

== system CSI_0313_4DC/AIP8/Subsystem5/PLL/Pos&Neg seq extract in subsystem  ==
  RIZ : Inport
  ffc : Inport  Port=2
  Add1 : Sum
  Add2 : Sum  Inputs=-+
  Demux1 : Demux  Outputs=3
  Gain{1..4} (4 alike) : Gain  Gain=0.5
  Ground : Ground
  Ground1 : Ground
  IIR_BPF_Im : MATLAB Function  TreatAsAtomicUnit=on  mask{fQ=fQ, fTs=fTs, iMode=IIR2 used as BPF in SOGI}
      mask prompts: fQ "Quality factor"; fTs "Sample time [s]"; iMode "Modes of 2nd-order transfer function"
  IIR_BPF_Re1 : MATLAB Function  TreatAsAtomicUnit=on  mask{fQ=fQ, fTs=fTs, iMode=IIR2 used as BPF in SOGI}
      mask prompts: fQ "Quality factor"; fTs "Sample time [s]"; iMode "Modes of 2nd-order transfer function"
  IIR_LPF_Im : MATLAB Function  TreatAsAtomicUnit=on  mask{fQ=fQ, fTs=fTs, iMode=IIR2 used as LPF in SOGI}
      mask prompts: fQ "Quality factor"; fTs "Sample time [s]"; iMode "Modes of 2nd-order transfer function"
  IIR_LPF_Re1 : MATLAB Function  TreatAsAtomicUnit=on  mask{fQ=fQ, fTs=fTs, iMode=IIR2 used as LPF in SOGI}
      mask prompts: fQ "Quality factor"; fTs "Sample time [s]"; iMode "Modes of 2nd-order transfer function"
  Mux : Mux  Inputs=3
  Mux1 : Mux  Inputs=3
  Mux2 : Mux
  Subtract1 : Sum  Inputs=+-
  Subtract2 : Sum
  Terminator : Terminator
  RizPos : Outport  VectorParamsAs1DForOutWhenUnconnected=on
  RizNeg : Outport  Port=2  VectorParamsAs1DForOutWhenUnconnected=on
  chk : Outport  Port=3  VectorParamsAs1DForOutWhenUnconnected=on
  wires:
  [ImBP] -> Add2/2
  [ffc] -> IIR_BPF_Im/2(fn)
  Add1/1 -> Gain3/1
  [ReLP] -> Mux2/3
  [ImBP] -> Mux2/4
  Demux1/1 -> [Re]
  RIZ/1 -> [Riz]
  Ground1/1 -> Mux1/3
  [ImLP] -> Mux2/2
  Add2/1 -> Gain4/1
  [ImLP] -> Subtract1/2
  [ReLP] -> Add1/1
  [ReBP] -> Subtract2/1
  [ImBP] -> Add1/2
  Gain1/1 -> [ReNeg]
  IIR_LPF_Re1/1(y) -> [ReLP]
  [Re] -> IIR_BPF_Re1/1(u)
  [RePos] -> Mux/1
  [ReBP] -> Subtract1/1
  Mux/1 -> RizPos/1
  [ffc] -> IIR_BPF_Re1/2(fn)
  Mux1/1 -> RizNeg/1
  IIR_BPF_Im/1(y) -> [ImBP]
  [Im] -> IIR_BPF_Im/1(u)
  Demux1/3 -> Terminator/1
  IIR_BPF_Re1/1(y) -> [ReBP]
  Gain3/1 -> [ImPos]
  IIR_LPF_Im/1(y) -> [ImLP]
  [ImNeg] -> Mux1/2
  [Im] -> IIR_LPF_Im/1(u)
  [ffc] -> IIR_LPF_Im/2(fn)
  [ImLP] -> Subtract2/2
  Demux1/2 -> [Im]
  Subtract1/1 -> Gain2/1
  [Re] -> IIR_LPF_Re1/1(u)
  [ffc] -> IIR_LPF_Re1/2(fn)
  [ReBP] -> Mux2/1
  [Riz] -> Demux1/1
  Ground/1 -> Mux/3
  [ReNeg] -> Mux1/1
  Mux2/1 -> chk/1
  Gain4/1 -> [ImNeg]
  Subtract2/1 -> Gain1/1
  Gain2/1 -> [RePos]
  [ReLP] -> Add2/1
  ffc/1 -> [ffc]
  [ImPos] -> Mux/2

== system CSI_0313_4DC/AIP9/Subsystem5/PLL/Pos&Neg seq extract in subsystem  ==
  RIZ : Inport
  ffc : Inport  Port=2
  Add1 : Sum
  Add2 : Sum  Inputs=-+
  Demux1 : Demux  Outputs=3
  Gain{1..4} (4 alike) : Gain  Gain=0.5
  Ground : Ground
  Ground1 : Ground
  IIR_BPF_Im : MATLAB Function  TreatAsAtomicUnit=on  mask{fQ=fQ, fTs=fTs, iMode=IIR2 used as BPF in SOGI}
      mask prompts: fQ "Quality factor"; fTs "Sample time [s]"; iMode "Modes of 2nd-order transfer function"
  IIR_BPF_Re1 : MATLAB Function  TreatAsAtomicUnit=on  mask{fQ=fQ, fTs=fTs, iMode=IIR2 used as BPF in SOGI}
      mask prompts: fQ "Quality factor"; fTs "Sample time [s]"; iMode "Modes of 2nd-order transfer function"
  IIR_LPF_Im : MATLAB Function  TreatAsAtomicUnit=on  mask{fQ=fQ, fTs=fTs, iMode=IIR2 used as LPF in SOGI}
      mask prompts: fQ "Quality factor"; fTs "Sample time [s]"; iMode "Modes of 2nd-order transfer function"
  IIR_LPF_Re1 : MATLAB Function  TreatAsAtomicUnit=on  mask{fQ=fQ, fTs=fTs, iMode=IIR2 used as LPF in SOGI}
      mask prompts: fQ "Quality factor"; fTs "Sample time [s]"; iMode "Modes of 2nd-order transfer function"
  Mux : Mux  Inputs=3
  Mux1 : Mux  Inputs=3
  Mux2 : Mux
  Subtract1 : Sum  Inputs=+-
  Subtract2 : Sum
  Terminator : Terminator
  RizPos : Outport  VectorParamsAs1DForOutWhenUnconnected=on
  RizNeg : Outport  Port=2  VectorParamsAs1DForOutWhenUnconnected=on
  chk : Outport  Port=3  VectorParamsAs1DForOutWhenUnconnected=on
  wires:
  [ImPos] -> Mux/2
  ffc/1 -> [ffc]
  [ReLP] -> Add2/1
  Gain2/1 -> [RePos]
  Subtract2/1 -> Gain1/1
  Gain4/1 -> [ImNeg]
  Mux2/1 -> chk/1
  [ReNeg] -> Mux1/1
  Ground/1 -> Mux/3
  [Riz] -> Demux1/1
  [ReBP] -> Mux2/1
  [ffc] -> IIR_LPF_Re1/2(fn)
  [Re] -> IIR_LPF_Re1/1(u)
  Subtract1/1 -> Gain2/1
  Demux1/2 -> [Im]
  [ImLP] -> Subtract2/2
  [ffc] -> IIR_LPF_Im/2(fn)
  [Im] -> IIR_LPF_Im/1(u)
  [ImNeg] -> Mux1/2
  IIR_LPF_Im/1(y) -> [ImLP]
  Gain3/1 -> [ImPos]
  IIR_BPF_Re1/1(y) -> [ReBP]
  Demux1/3 -> Terminator/1
  [Im] -> IIR_BPF_Im/1(u)
  IIR_BPF_Im/1(y) -> [ImBP]
  Mux1/1 -> RizNeg/1
  [ffc] -> IIR_BPF_Re1/2(fn)
  Mux/1 -> RizPos/1
  [ReBP] -> Subtract1/1
  [RePos] -> Mux/1
  [Re] -> IIR_BPF_Re1/1(u)
  IIR_LPF_Re1/1(y) -> [ReLP]
  Gain1/1 -> [ReNeg]
  [ImBP] -> Add1/2
  [ReBP] -> Subtract2/1
  [ReLP] -> Add1/1
  [ImLP] -> Subtract1/2
  Add2/1 -> Gain4/1
  [ImLP] -> Mux2/2
  Ground1/1 -> Mux1/3
  RIZ/1 -> [Riz]
  Demux1/1 -> [Re]
  [ImBP] -> Mux2/4
  [ReLP] -> Mux2/3
  Add1/1 -> Gain3/1
  [ffc] -> IIR_BPF_Im/2(fn)
  [ImBP] -> Add2/2

== matlab function CSI_0313_4DC/AIP1/SPWM_Three Level/Voltage update timing generator1 ==
  data: Trigger input; Tupdate output; Update input
function Tupdate = fcn(Trigger,Update)
    persistent cntx Tupdate1;
    if isempty(cntx)
         if(Update == 1)
            cntx =  1;
         else
            cntx =  3;
         end
        Tupdate1 = 0;
    end
    
    if(Trigger > 0)
        cntx = cntx +1;
    else
        cntx = cntx;
    end
    
    
    if(Trigger > 0 && cntx == 2)
        Tupdate1 = Trigger;
    else
        Tupdate1 = 0;        
    end
    if(cntx == 2*Update)
        cntx = 0;
    end

    Tupdate = Tupdate1;

== matlab function CSI_0313_4DC/AIP3/SPWM_Three Level/Carrier Gen ==
  data: carrier output; sgn output; fdelt parameter; fsw input size=1
function [carrier, sgn] = fcn(fdelt, fsw)

persistent waveSaw stage;
if isempty(waveSaw)
    waveSaw = 0;
    stage = 0;
end

fHtop = 1/fdelt;
fHalf = 0.5*fHtop;
if (waveSaw < fHalf)
    waveTri = waveSaw;
else
    waveTri = fHtop - waveSaw;
end
sgn = 1-stage;
if (waveSaw < (fHalf-0.5*fsw))
    stage = 1;
elseif (waveSaw < (fHtop-0.5*fsw))
    sgn = stage;
    stage = 0;
else
	stage = 1;
end
	waveSaw = waveSaw + fsw;
if (waveSaw >= fHtop)
    waveSaw = waveSaw - fHtop;
end

carrier = waveTri / fHalf;

end

== matlab function CSI_0313_4DC/AIP3/SPWM_Three Level/Pulse Modulation ==
  data: carrier input; Pulse output; sgn input; update input; mod input; chk output; chk1 output
function [Pulse,chk,chk1] = fcn(carrier, sgn, update, mod)

persistent intx cnt;
if isempty(intx)
    intx = zeros(3,1);
    ref = zeros(3,1);    
    cnt = zeros(3,1);
end

Gate = zeros(3,4);
carrier_up = carrier;
carrier_down = carrier-1;

for i=1:1:3
    if(update > 0)
        ref(i) = mod(i);
        cnt(i) = 0;
    else
        ref(i) = intx(i);        
    end    
    intx(i) = ref(i);
    %Limitter
    if(ref(i) > 0.99)   
        ref(i) = 0.99;
    elseif(ref(i) < -0.99)
        ref(i) = -0.99;
    end
%%%%%%%%%%%    
end

for i=1:1:3
    if (ref(i) >= carrier_up)
       Gate(i,1) = 1;
       Gate(i,3) = 0;
    elseif (ref(i) <= carrier_up)
       Gate(i,1) = 0;
       Gate(i,3) = 1;
    end
    
    if (ref(i) >= carrier_down)
       Gate(i,2) = 1;
       Gate(i,4) = 0;
    elseif (ref(i) <= carrier_down)
       Gate(i,2) = 0;
       Gate(i,4) = 1;
    end
end
 
Pulse = [Gate(1,:), Gate(2,:),Gate(3,:)];
chk = Gate(1,:) ;
chk1 = ref(1) ;

end

== matlab function CSI_0313_4DC/AIP1/Subsystem7/ABC_To_RIZ1 ==
  data: ABC input; RIZ output
function RIZ = ABC_To_RIZ(ABC)
    % Clarke Transfer from ABC axis to Re-Im axis
    RIZ = [0;0;0];
    RIZ(1) = (2*ABC(1)-ABC(2)-ABC(3))/3;
    RIZ(2) = sqrt(3)*(ABC(2)-ABC(3))/3;
    RIZ(3) = (ABC(1)+ABC(2)+ABC(3))/3;
end

== matlab function CSI_0313_4DC/AIP2/SPWM_Three Level/Carrier Gen ==
  data: carrier output; sgn output; fdelt parameter; fsw input size=1
function [carrier, sgn] = fcn(fdelt, fsw)

persistent waveSaw stage;
if isempty(waveSaw)
    waveSaw = 0;
    stage = 0;
end

fHtop = 1/fdelt;
fHalf = 0.5*fHtop;
if (waveSaw < fHalf)
    waveTri = waveSaw;
else
    waveTri = fHtop - waveSaw;
end
sgn = 1-stage;
if (waveSaw < (fHalf-0.5*fsw))
    stage = 1;
elseif (waveSaw < (fHtop-0.5*fsw))
    sgn = stage;
    stage = 0;
else
	stage = 1;
end
	waveSaw = waveSaw + fsw;
if (waveSaw >= fHtop)
    waveSaw = waveSaw - fHtop;
end

carrier = waveTri / fHalf;

end

== matlab function CSI_0313_4DC/AIP2/SPWM_Three Level/Pulse Modulation ==
  data: carrier input; Pulse output; sgn input; update input; mod input; chk output; chk1 output
function [Pulse,chk,chk1] = fcn(carrier, sgn, update, mod)

persistent intx cnt;
if isempty(intx)
    intx = zeros(3,1);
    ref = zeros(3,1);    
    cnt = zeros(3,1);
end

Gate = zeros(3,4);
carrier_up = carrier;
carrier_down = carrier-1;

for i=1:1:3
    if(update > 0)
        ref(i) = mod(i);
        cnt(i) = 0;
    else
        ref(i) = intx(i);        
    end    
    intx(i) = ref(i);
    %Limitter
    if(ref(i) > 0.99)   
        ref(i) = 0.99;
    elseif(ref(i) < -0.99)
        ref(i) = -0.99;
    end
%%%%%%%%%%%    
end

for i=1:1:3
    if (ref(i) >= carrier_up)
       Gate(i,1) = 1;
       Gate(i,3) = 0;
    elseif (ref(i) <= carrier_up)
       Gate(i,1) = 0;
       Gate(i,3) = 1;
    end
    
    if (ref(i) >= carrier_down)
       Gate(i,2) = 1;
       Gate(i,4) = 0;
    elseif (ref(i) <= carrier_down)
       Gate(i,2) = 0;
       Gate(i,4) = 1;
    end
end
 
Pulse = [Gate(1,:), Gate(2,:),Gate(3,:)];
chk = Gate(1,:) ;
chk1 = ref(1) ;

end

== matlab function CSI_0313_4DC/AIP2/SPWM_Three Level/Tdt Insert ==
  data: Gate output; pulse input; tdt parameter; fdelt parameter; st input; chk output
function [Gate, chk] = fcn(pulse, tdt, fdelt, st)

persistent intx cnt;
if isempty(intx)
    intx = zeros(12,1);
    cnt = zeros(12,1);
end
Gate = pulse;

for i=1:1:12
    if( (Gate(i)==1) && (intx(i)==0) )
			cnt(i) = cnt(i)+fdelt;
			if (cnt(i) >= tdt)
				Gate(i) = 1;
				intx(i) = 1;
				cnt(i) = 0;
			else
				Gate(i) = intx(i);
            end
    else
			intx(i) = Gate(i);
			cnt(i)  = 0;
    end
    if(st == 0)
    	Gate(i) = 0;
    end
end
chk = Gate;

end

== matlab function CSI_0313_4DC/AIP2/SPWM_Three Level/Voltage update timing generator ==
  data: Trigger input; Tupdate output; Update input
function Tupdate = fcn(Trigger,Update)
    persistent cntx Tupdate1;
    if isempty(cntx)
        cntx = 2*Update-1;
        Tupdate1 = 0;
    end
    
    if(Trigger > 0)
        cntx = cntx +1;
    else
        cntx = cntx;
    end
    
    
    if(Trigger > 0 && cntx == 4)
        Tupdate1 = Trigger;
    else
        Tupdate1 = 0;        
    end
    if(cntx == 2*Update)
        cntx = 0;
    end

    Tupdate = Tupdate1;

== matlab function CSI_0313_4DC/AIP2/SPWM_Three Level/Voltage update timing generator1 ==
  data: Trigger input; Tupdate output; Update input
function Tupdate = fcn(Trigger,Update)
    persistent cntx Tupdate1;
    if isempty(cntx)
         if(Update == 1)
            cntx =  1;
         else
            cntx =  3;
         end
        Tupdate1 = 0;
    end
    
    if(Trigger > 0)
        cntx = cntx +1;
    else
        cntx = cntx;
    end
    
    
    if(Trigger > 0 && cntx == 2)
        Tupdate1 = Trigger;
    else
        Tupdate1 = 0;        
    end
    if(cntx == 2*Update)
        cntx = 0;
    end

    Tupdate = Tupdate1;

== matlab function CSI_0313_4DC/AIP2/Sample//Moving window5 ==
  data: yout output; uin input; trig input; iNumAvg parameter; iNumDly parameter; ubase parameter
function yout=sample(uin,trig,iNumAvg,iNumDly,ubase)

persistent uary cnt sum yavg;

iNumIn = length(uin);
iNumDly = iNumDly+1;
if isempty(cnt)  
    cnt = 0;
    uary = zeros(iNumIn,iNumAvg);
    sum = zeros(iNumIn,1);
    yavg = zeros(iNumIn,iNumDly);    
end

if(trig >0) 
    for i=1:1:iNumIn
        for j=iNumDly:-1:2
            yavg(i,j)= yavg(i,j-1);
        end
    end
    cnt = cnt +1;
    for i=1:1:iNumIn
        uary(i,cnt) = uin(i)/ubase;
        sum(i) = sum(i)+uary(i,cnt);
    end
    if(cnt == iNumAvg)
        cnt = 0;
        for i=1:1:iNumIn
            yavg(i,1)=sum(i)/iNumAvg;
        end
        for i=1:1:iNumIn
            sum(i)=0;
        end
    end        
end
    yout = yavg(:,iNumDly);
end

== matlab function CSI_0313_4DC/AIP3/SPWM_Three Level/Tdt Insert ==
  data: Gate output; pulse input; tdt parameter; fdelt parameter; st input; chk output
function [Gate, chk] = fcn(pulse, tdt, fdelt, st)

persistent intx cnt;
if isempty(intx)
    intx = zeros(12,1);
    cnt = zeros(12,1);
end
Gate = pulse;

for i=1:1:12
    if( (Gate(i)==1) && (intx(i)==0) )
			cnt(i) = cnt(i)+fdelt;
			if (cnt(i) >= tdt)
				Gate(i) = 1;
				intx(i) = 1;
				cnt(i) = 0;
			else
				Gate(i) = intx(i);
            end
    else
			intx(i) = Gate(i);
			cnt(i)  = 0;
    end
    if(st == 0)
    	Gate(i) = 0;
    end
end
chk = Gate;

end

== matlab function CSI_0313_4DC/AIP3/SPWM_Three Level/Voltage update timing generator ==
  data: Trigger input; Tupdate output; Update input
function Tupdate = fcn(Trigger,Update)
    persistent cntx Tupdate1;
    if isempty(cntx)
        cntx = 2*Update-1;
        Tupdate1 = 0;
    end
    
    if(Trigger > 0)
        cntx = cntx +1;
    else
        cntx = cntx;
    end
    
    
    if(Trigger > 0 && cntx == 4)
        Tupdate1 = Trigger;
    else
        Tupdate1 = 0;        
    end
    if(cntx == 2*Update)
        cntx = 0;
    end

    Tupdate = Tupdate1;

== matlab function CSI_0313_4DC/AIP3/SPWM_Three Level/Voltage update timing generator1 ==
  data: Trigger input; Tupdate output; Update input
function Tupdate = fcn(Trigger,Update)
    persistent cntx Tupdate1;
    if isempty(cntx)
         if(Update == 1)
            cntx =  1;
         else
            cntx =  3;
         end
        Tupdate1 = 0;
    end
    
    if(Trigger > 0)
        cntx = cntx +1;
    else
        cntx = cntx;
    end
    
    
    if(Trigger > 0 && cntx == 2)
        Tupdate1 = Trigger;
    else
        Tupdate1 = 0;        
    end
    if(cntx == 2*Update)
        cntx = 0;
    end

    Tupdate = Tupdate1;

== matlab function CSI_0313_4DC/AIP3/Sample//Moving window5 ==
  data: yout output; uin input; trig input; iNumAvg parameter; iNumDly parameter; ubase parameter
function yout=sample(uin,trig,iNumAvg,iNumDly,ubase)

persistent uary cnt sum yavg;

iNumIn = length(uin);
iNumDly = iNumDly+1;
if isempty(cnt)  
    cnt = 0;
    uary = zeros(iNumIn,iNumAvg);
    sum = zeros(iNumIn,1);
    yavg = zeros(iNumIn,iNumDly);    
end

if(trig >0) 
    for i=1:1:iNumIn
        for j=iNumDly:-1:2
            yavg(i,j)= yavg(i,j-1);
        end
    end
    cnt = cnt +1;
    for i=1:1:iNumIn
        uary(i,cnt) = uin(i)/ubase;
        sum(i) = sum(i)+uary(i,cnt);
    end
    if(cnt == iNumAvg)
        cnt = 0;
        for i=1:1:iNumIn
            yavg(i,1)=sum(i)/iNumAvg;
        end
        for i=1:1:iNumIn
            sum(i)=0;
        end
    end        
end
    yout = yavg(:,iNumDly);
end

== matlab function CSI_0313_4DC/AIP2/Subsystem7/Pos Compensation1/PI Ctrl2 ==
  data: err input; y output; fKI parameter; fMinLmt parameter; fTs parameter; fMaxLmt parameter; fKP parameter
function y = PICtrl(err, fKI, fMinLmt, fTs, fMaxLmt, fKP)
    % y[n] = y[n-1] + KP*(x[n]-x[n-1]) + (KP*KI*TS*0.5)*(x[n]+x[n-1])
    % err:  error input
    % fKP:   Proportional gain
    % fKI:   Integral Coefficient
    % fMinLmt: Minimum limitation
    % fMaxLmt: Maximum limitation
    % fTs:  Sampling time
    
    % t(1,2) stores x[n],x[n-1]; t(2,2) stores y[n],y[n-1]
    persistent t;      
    if isempty(t)           % Initialization
        t = zeros(2,2);
    end
    
%     if(Trig > 0)
        t(1,1) = err;
        t(2,1) = t(2,2) + fKP*(t(1,1)-t(1,2)) + fKP*fKI*0.5*(t(1,1)+t(1,2))*fTs;   
    
        if (t(2,1) < fMinLmt)
            t(2,1) = fMinLmt;
        elseif (t(2,1) > fMaxLmt)
            t(2,1) = fMaxLmt;
        end
    
        t(1,2) = t(1,1);
        t(2,2) = t(2,1);
%     else
%         t(1,1) = t(1,1);
%         t(2,1) = t(2,1);      
%         t(1,2) = t(1,2);
%         t(2,2) = t(2,2);
%     end
    y = t(2,1);
end

== matlab function CSI_0313_4DC/AIP3/Subsystem7/Pos Compensation1/PI Ctrl2 ==
  data: err input; y output; fKI parameter; fMinLmt parameter; fTs parameter; fMaxLmt parameter; fKP parameter
function y = PICtrl(err, fKI, fMinLmt, fTs, fMaxLmt, fKP)
    % y[n] = y[n-1] + KP*(x[n]-x[n-1]) + (KP*KI*TS*0.5)*(x[n]+x[n-1])
    % err:  error input
    % fKP:   Proportional gain
    % fKI:   Integral Coefficient
    % fMinLmt: Minimum limitation
    % fMaxLmt: Maximum limitation
    % fTs:  Sampling time
    
    % t(1,2) stores x[n],x[n-1]; t(2,2) stores y[n],y[n-1]
    persistent t;      
    if isempty(t)           % Initialization
        t = zeros(2,2);
    end
    
%     if(Trig > 0)
        t(1,1) = err;
        t(2,1) = t(2,2) + fKP*(t(1,1)-t(1,2)) + fKP*fKI*0.5*(t(1,1)+t(1,2))*fTs;   
    
        if (t(2,1) < fMinLmt)
            t(2,1) = fMinLmt;
        elseif (t(2,1) > fMaxLmt)
            t(2,1) = fMaxLmt;
        end
    
        t(1,2) = t(1,1);
        t(2,2) = t(2,1);
%     else
%         t(1,1) = t(1,1);
%         t(2,1) = t(2,1);      
%         t(1,2) = t(1,2);
%         t(2,2) = t(2,2);
%     end
    y = t(2,1);
end

== matlab function CSI_0313_4DC/AIP4/Subsystem7/Pos Compensation1/PI Ctrl2 ==
  data: err input; y output; fKI parameter; fMinLmt parameter; fTs parameter; fMaxLmt parameter; fKP parameter
function y = PICtrl(err, fKI, fMinLmt, fTs, fMaxLmt, fKP)
    % y[n] = y[n-1] + KP*(x[n]-x[n-1]) + (KP*KI*TS*0.5)*(x[n]+x[n-1])
    % err:  error input
    % fKP:   Proportional gain
    % fKI:   Integral Coefficient
    % fMinLmt: Minimum limitation
    % fMaxLmt: Maximum limitation
    % fTs:  Sampling time
    
    % t(1,2) stores x[n],x[n-1]; t(2,2) stores y[n],y[n-1]
    persistent t;      
    if isempty(t)           % Initialization
        t = zeros(2,2);
    end
    
%     if(Trig > 0)
        t(1,1) = err;
        t(2,1) = t(2,2) + fKP*(t(1,1)-t(1,2)) + fKP*fKI*0.5*(t(1,1)+t(1,2))*fTs;   
    
        if (t(2,1) < fMinLmt)
            t(2,1) = fMinLmt;
        elseif (t(2,1) > fMaxLmt)
            t(2,1) = fMaxLmt;
        end
    
        t(1,2) = t(1,1);
        t(2,2) = t(2,1);
%     else
%         t(1,1) = t(1,1);
%         t(2,1) = t(2,1);      
%         t(1,2) = t(1,2);
%         t(2,2) = t(2,2);
%     end
    y = t(2,1);
end

== matlab function CSI_0313_4DC/AIP5/Subsystem7/Pos Compensation1/PI Ctrl2 ==
  data: err input; y output; fKI parameter; fMinLmt parameter; fTs parameter; fMaxLmt parameter; fKP parameter
function y = PICtrl(err, fKI, fMinLmt, fTs, fMaxLmt, fKP)
    % y[n] = y[n-1] + KP*(x[n]-x[n-1]) + (KP*KI*TS*0.5)*(x[n]+x[n-1])
    % err:  error input
    % fKP:   Proportional gain
    % fKI:   Integral Coefficient
    % fMinLmt: Minimum limitation
    % fMaxLmt: Maximum limitation
    % fTs:  Sampling time
    
    % t(1,2) stores x[n],x[n-1]; t(2,2) stores y[n],y[n-1]
    persistent t;      
    if isempty(t)           % Initialization
        t = zeros(2,2);
    end
    
%     if(Trig > 0)
        t(1,1) = err;
        t(2,1) = t(2,2) + fKP*(t(1,1)-t(1,2)) + fKP*fKI*0.5*(t(1,1)+t(1,2))*fTs;   
    
        if (t(2,1) < fMinLmt)
            t(2,1) = fMinLmt;
        elseif (t(2,1) > fMaxLmt)
            t(2,1) = fMaxLmt;
        end
    
        t(1,2) = t(1,1);
        t(2,2) = t(2,1);
%     else
%         t(1,1) = t(1,1);
%         t(2,1) = t(2,1);      
%         t(1,2) = t(1,2);
%         t(2,2) = t(2,2);
%     end
    y = t(2,1);
end

== matlab function CSI_0313_4DC/AIP2/Subsystem3/IIR_1st1 ==
  data: u input; fc parameter; y output; fTs parameter
function y = IIR_1st(u, fc, fTs)
    % y[n] = (-(1-T)*y[n-1] + x[n] + x[n-1])/(1+T)
    % u:    Input
    % fc:   Cut-off frequency
    % fTs:  Sample time
    
    persistent t;
    
    if isempty(t)
        t = zeros(2,2);
    end
    
    T = 1/(pi*fc*fTs);            
    
%     if(Trig > 0)
        t(1,1) = u;        
        t(2,1) = (t(1,1) + t(1,2) - (1-T)*t(2,2)) / (1+T);
    
        t(1,2) = t(1,1);
        t(2,2) = t(2,1);
%     else
%         t(1,1) = t(1,1);        
%         t(2,1) = t(2,1);
%     
%         t(1,2) = t(1,2);
%         t(2,2) = t(2,2);
%     end
%     
    y = t(2,1);
end

== matlab function CSI_0313_4DC/Programmal Grid/Programmal Grid  ==
  data: ua output; ub output; uc output; Tdelt parameter; K5 parameter; K7 parameter; K21 parameter; K120 parameter; t input
function [ua, ub, uc] = fcn(Tdelt,K5, K7, K21,K120,t)
persistent theta; 
 % Initialization
 if isempty(theta)           
    theta = pi/2;
 end 

f = 50;
Vm = 400*sqrt(2/3);
Tflt = 0.2;             %% fault duration time[s]
Vsag = 0.05 * Vm;        %% voltage level configuration during the fault
theta = theta + 2*pi*f*Tdelt;
if(theta >= 2*pi)
    theta = theta-2*pi;
end

Tinrpt = 12.21;
if (t < Tinrpt)
    Vol = Vm;
elseif (t>=Tinrpt && t<(Tinrpt+0.004))  %% the fault starts and ends in 4ms
    Vol = Vm-(t-Tinrpt)*(Vm - Vsag)/0.004;
elseif (t>=Tinrpt && t<(Tinrpt+0.004+Tflt)) %% the fault sustain Tflt[s]
    Vol = Vsag;
elseif (t>=(Tinrpt+0.004+Tflt) && t< (Tinrpt+0.008+Tflt))  %% the fault recoverys in 4ms
    Vol = Vsag+(t-(Tinrpt+0.004+Tflt))*(Vm - Vsag)/0.004;
else
    Vol = Vm;
end

ua = Vol*sin(theta)+K5*Vm*sin(5.0*theta)+K7*Vm*sin(7.0*theta)+K21*Vm*sin(21.0*theta)+K120*Vm*sin(120.0*theta);
ub = Vol*sin(theta-2*pi/3)+K5*Vm*sin(5.0*(theta-2*pi/3))+K7*Vm*sin(7.0*(theta-2*pi/3))+K120*Vm*sin(120.0*(theta-2*pi/3));
uc = Vol*sin(theta+2*pi/3)+K5*Vm*sin(5.0*(theta+2*pi/3))+K7*Vm*sin(7.0*(theta+2*pi/3))+K120*Vm*sin(120.0*(theta+2*pi/3));

end

== matlab function CSI_0313_4DC/AIP2/Subsystem5/PLL/ABC_To_RIZ ==
  data: ABC input size=3; RIZ output size=3
function RIZ = ABC_To_RIZ(ABC)
    % Clarke Transfer from ABC axis to Re-Im axis
    RIZ = [0;0;0];
    RIZ(1) = (2*ABC(1)-ABC(2)-ABC(3))/3;
    RIZ(2) = sqrt(3)*(ABC(2)-ABC(3))/3;
    RIZ(3) = (ABC(1)+ABC(2)+ABC(3))/3;
end
